simulink model "Modelo_GuPu"  (Simulink 9.3)
settings: Solver=ode45  StartTime=0.0  StopTime=1000  MaxStep=0.1  RelTol=1e-6  EnableMultiTasking=on
settings Model: Creator=Marcelo  LastModifiedBy=Rick Sanchez
settings DataIOCC: SaveOutput=off  SignalLoggingName=sigsOut
settings OptimizationCC: BlockReduction=off  BooleanDataType=off  ExpressionDepthLimit=2147483647
settings DebuggingCC: SaveWithParameterizedLinksMsg=none  SignalResolutionControl=TryResolveAllWithWarning  MultiTaskDSMMsg=warning  MultiTaskCondExecSysMsg=none  StateNameClashWarn=warning
settings HardwareCC: TargetUnknown=on
settings GRTTargetCC: GeneratePreprocessorConditionals=Disable all

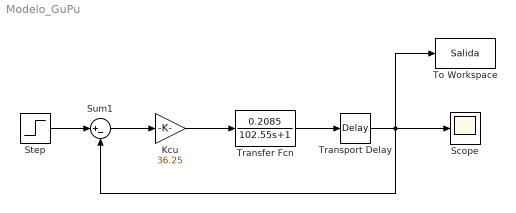
== system Modelo_GuPu ==
  Kcu : Gain  Gain=36.25
  Scope : Scope
  Step : Step  Time=50  Before=1  SampleTime=0
  Sum1 : Sum  Inputs=|+-  SaturateOnIntegerOverflow=on  InputSameDT=on  OutDataTypeStr=Inherit: Same as first input
  To Workspace : ToWorkspace  VariableName=Salida
  Transfer Fcn : TransferFcn  Numerator=[0.2085]  Denominator=[102.55 1]
  Transport Delay : TransportDelay  DelayTime=23.3
  wires:
  Transfer Fcn/1 -> Transport Delay/1
  Transport Delay/1 -> To Workspace/1, Scope/1, Sum1/2
  Kcu/1 -> Transfer Fcn/1
  Sum1/1 -> Kcu/1
  Step/1 -> Sum1/1
